simulink model "ponto5"  (R2018a)
settings: Solver=VariableStepAuto  StartTime=0.0  StopTime=100  RelTol=1e-3
values from neighbouring files (symbols this model uses):
  aa0 = 5.27*deg    (= 0.0919788515801)    [tb30.m]
  ah = [xu xw -aa0*u0 -g*cos(tt0) 0 ... (first row only)    [tb30.m]
  bh = [xde xdt; zde 0; mde+mwp*zde mdt; 0 0; 0 0]    [tb30.m]
  deg = pi/180    (= 0.0174532925199)    [tb30.m]
  f = ([1 0 0 0 0;0 0 0 0 1]*g)^-1    [tb30.m]
  ft = 0.3048    [tb30.m]
  k2 = lqr(ah,bh,q,r)    [tb30.m]
  ms = 0.514444444    [tb30.m]
  u0 = 85.4*ms    (= 43.9335555176)    [tb30.m]
libraries: simulink x3
settings Model: Creator=inespassinhas  LastModifiedBy=rafae
settings CodeAppCC: StateflowObjectComments=on

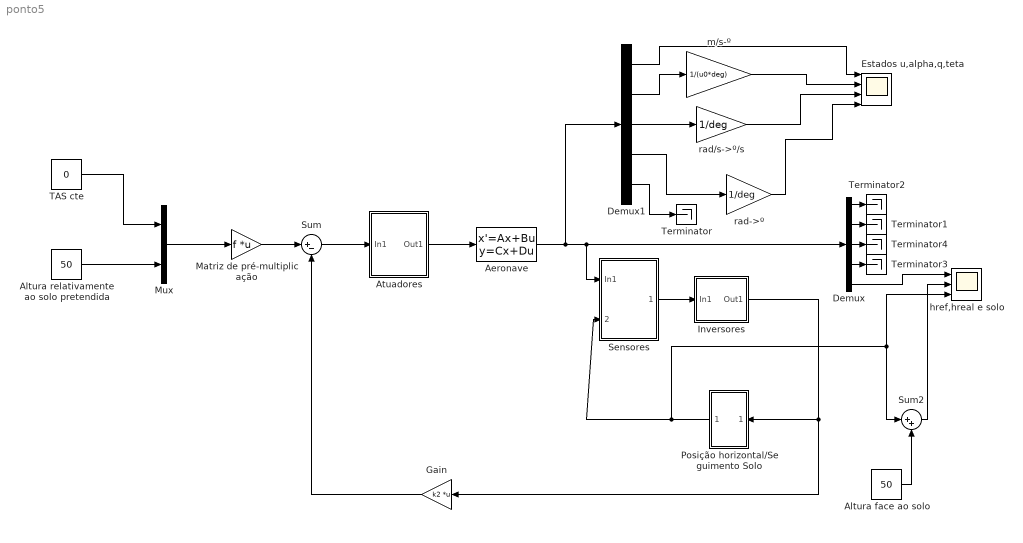
== system ponto5 ==
  Aeronave : StateSpace  A=ah  B=bh  C=eye(5)  D=zeros(5,2)  InitialCondition=[0 0 0 0 50+5*u0]
  "Altura face ao solo   " : Constant  Value=50
  Altura relativamente ao solo pretendida : Constant  Value=50
  Atuadores : Subsystem
  Demux : Demux  Outputs=5
  Demux1 : Demux  Outputs=5
  Estados u,alpha,q,teta : Scope  NumInputPorts=4
  Gain : Gain  Gain=k2  Multiplication=Matrix(K*u)
  Inversores : Subsystem
  Matriz de pré-multiplicação : Gain  Gain=f  Multiplication=Matrix(K*u)
  Mux : Mux  Inputs=2
  Posição horizontal/Seguimento Solo : Subsystem
  Sensores : Subsystem
  Sum : Sum  Inputs=|+-
  Sum2 : Sum  Inputs=|++
  TAS cte : Constant  Value=0
  Terminator{,1..4} (5 alike) : Terminator
  href,hreal e solo : Scope  NumInputPorts=3
  m/s-º : Gain  Gain=1/(u0*deg)
  rad->º : Gain  Gain=1/deg
  rad/s->º/s : Gain  Gain=1/deg
  wires:
  Gain/1 -> Sum/2
  Aeronave/1 -> Sensores/1(In1), Demux/1, Demux1/1
  Mux/1 -> Matriz de pré-multiplicação/1
  Matriz de pré-multiplicação/1 -> Sum/1
  Sensores/1(Out1) -> Inversores/1(In1)
  Atuadores/1(Out1) -> Aeronave/1
  Sum/1 -> Atuadores/1(In1)
  TAS cte/1 -> Mux/1
  Altura relativamente ao solo pretendida/1 -> Mux/2
  Demux/5 -> href,hreal e solo/1
  Sum2/1 -> href,hreal e solo/2
  Inversores/1(Out1) -> Gain/1, Posição horizontal/Seguimento Solo/1(In1)
  Posição horizontal/Seguimento Solo/1(Out1) -> href,hreal e solo/3, Sum2/1, Sensores/2("altura do solo ")
  "Altura face ao solo   "/1 -> Sum2/2
  Demux1/1 -> Estados u,alpha,q,teta/1
  Demux1/2 -> m/s-º/1
  m/s-º/1 -> Estados u,alpha,q,teta/2
  Demux1/3 -> rad/s->º/s/1
  rad/s->º/s/1 -> Estados u,alpha,q,teta/3
  Demux1/4 -> rad->º/1
  rad->º/1 -> Estados u,alpha,q,teta/4
  Demux1/5 -> Terminator/1
  Demux/4 -> Terminator3/1
  Demux/1 -> Terminator2/1
  Demux/2 -> Terminator1/1
  Demux/3 -> Terminator4/1

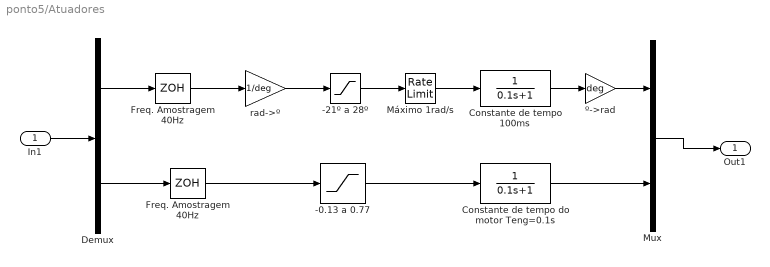
== system ponto5/Atuadores ==
  In1 : Inport
  " Constante de tempo do motor Teng=0.1s" : TransferFcn  Denominator=[0.1 1]
  -0.13 a 0.77 : Saturate  UpperLimit=0.77  LowerLimit=-0.13
  -21º a 28º : Saturate  UpperLimit=28  LowerLimit=-21
  Constante de tempo 100ms : TransferFcn  Denominator=[0.1 1]
  Demux : Demux  Outputs=2
  Freq. Amostragem 40Hz : ZeroOrderHold  SampleTime=1/40
  Freq. Amostragem 40Hz : ZeroOrderHold  SampleTime=1/40
  Mux : Mux  Inputs=2
  Máximo 1rad/s : RateLimiter  RisingSlewLimit=1/deg  FallingSlewLimit=-1/deg  SampleTimeMode=inherited
  rad->º : Gain  Gain=1/deg
  º->rad : Gain  Gain=deg
  Out1 : Outport
  wires:
  Mux/1 -> Out1/1
  In1/1 -> Demux/1
  Demux/2 -> Freq. Amostragem 40Hz/1
  Demux/1 -> Freq. Amostragem 40Hz/1
  Freq. Amostragem 40Hz/1 -> rad->º/1
  rad->º/1 -> -21º a 28º/1
  -21º a 28º/1 -> Máximo 1rad/s/1
  Máximo 1rad/s/1 -> Constante de tempo 100ms/1
  Constante de tempo 100ms/1 -> º->rad/1
  º->rad/1 -> Mux/1
  Freq. Amostragem 40Hz/1 -> -0.13 a 0.77/1
  -0.13 a 0.77/1 -> " Constante de tempo do motor Teng=0.1s"/1
  " Constante de tempo do motor Teng=0.1s"/1 -> Mux/2

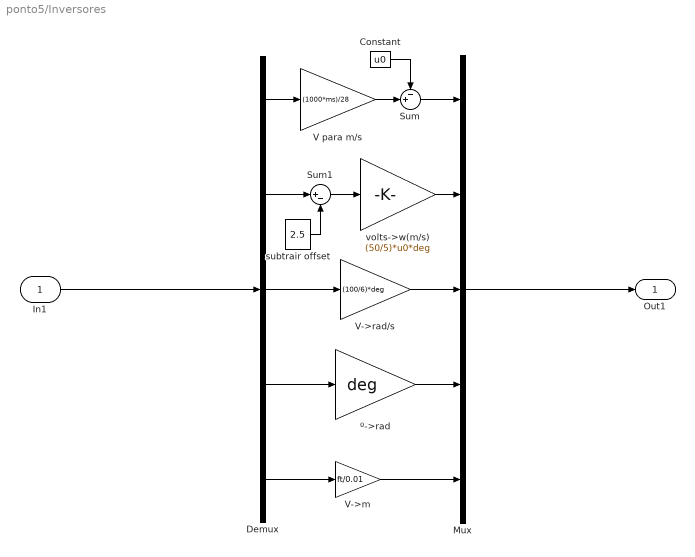
== system ponto5/Inversores ==
  In1 : Inport
  Constant : Constant  Value=u0
  Demux : Demux  Outputs=5
  Mux : Mux  Inputs=5
  Sum : Sum  Inputs=-+|
  Sum1 : Sum  Inputs=|+-
  V para m/s : Gain  Gain=(1000*ms)/28
  V->m : Gain  Gain=ft/0.01
  V->rad/s : Gain  Gain=(100/6)*deg
  subtrair offset : Constant  Value=2.5
  volts->w(m/s) : Gain  Gain=(50/5)*u0*deg
  º->rad : Gain  Gain=deg
  Out1 : Outport
  wires:
  In1/1 -> Demux/1
  Mux/1 -> Out1/1
  Demux/1 -> V para m/s/1
  V para m/s/1 -> Sum/2
  Constant/1 -> Sum/1
  Sum/1 -> Mux/1
  Demux/2 -> Sum1/1
  subtrair offset/1 -> Sum1/2
  Sum1/1 -> volts->w(m/s)/1
  volts->w(m/s)/1 -> Mux/2
  Demux/3 -> V->rad/s/1
  V->rad/s/1 -> Mux/3
  Demux/4 -> º->rad/1
  º->rad/1 -> Mux/4
  Demux/5 -> V->m/1
  V->m/1 -> Mux/5

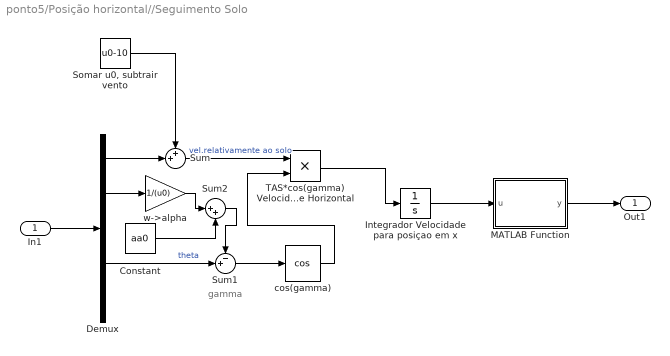
== system ponto5/Posição horizontal//Seguimento Solo ==
  note: gamma
  In1 : Inport
  Constant : Constant  Value=aa0
  Demux : Demux  Outputs=5
  Integrador Velocidade para posiçao em x : Integrator
  MATLAB Function : MATLAB Function  TreatAsAtomicUnit=on
  "Somar u0, subtrair vento" : Constant  Value=u0-10
  Sum : Sum  Inputs=++|
  Sum1 : Sum  Inputs=-+|
  Sum2 : Sum  Inputs=|++
  TAS*cos(gamma) Velocidade Horizontal : Product
  cos(gamma) : Trigonometry  Operator=cos
  w->alpha : Gain  Gain=1/(u0)
  Out1 : Outport
  wires:
  In1/1 -> Demux/1
  Demux/1 -> Sum/2
  "Somar u0, subtrair vento"/1 -> Sum/1
  Demux/2 -> w->alpha/1
  Demux/4 -> Sum1/2  "theta"
  Sum1/1 -> cos(gamma)/1
  cos(gamma)/1 -> TAS*cos(gamma) Velocidade Horizontal/2
  Sum/1 -> TAS*cos(gamma) Velocidade Horizontal/1  "vel.relativamente ao solo"
  TAS*cos(gamma) Velocidade Horizontal/1 -> Integrador Velocidade para posiçao em x/1
  Integrador Velocidade para posiçao em x/1 -> MATLAB Function/1(u)
  MATLAB Function/1(y) -> Out1/1
  Sum2/1 -> Sum1/1
  w->alpha/1 -> Sum2/1
  Constant/1 -> Sum2/2

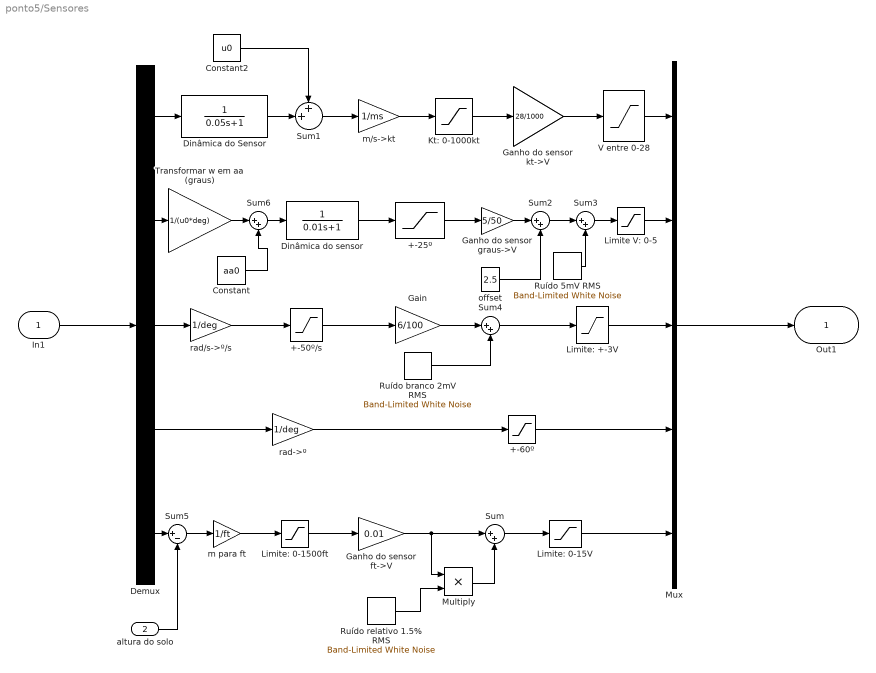
== system ponto5/Sensores ==
  In1 : Inport
  "altura do solo " : Inport  Port=2
  " Dinâmica do Sensor" : TransferFcn  Denominator=[0.05 1]
  +-25º : Saturate  UpperLimit=25  LowerLimit=-25
  +-50º/s : Saturate  UpperLimit=50  LowerLimit=-50
  +-60º : Saturate  UpperLimit=60  LowerLimit=-60
  Constant : Constant  Value=aa0
  Constant2 : Constant  Value=u0
  Demux : Demux  Outputs=5
  Dinâmica do sensor : TransferFcn  Denominator=[0.01 1]
  Gain : Gain  Gain=6/100
  Ganho do sensor ft->V : Gain  Gain=0.01
  Ganho do sensor graus->V : Gain  Gain=5/50
  Ganho do sensor kt->V : Gain  Gain=28/1000
  Kt: 0-1000kt : Saturate  UpperLimit=1000  LowerLimit=0
  Limite V: 0-5 : Saturate  UpperLimit=5  LowerLimit=0
  Limite: +-3V : Saturate  UpperLimit=3  LowerLimit=-3
  Limite: 0-1500ft : Saturate  UpperLimit=1500  LowerLimit=0
  Limite: 0-15V : Saturate  UpperLimit=1500*0.01  LowerLimit=0
  Multiply : Product
  Mux : Mux  Inputs=5
  Ruído 5mV RMS : simulink/Sources/Band-Limited White Noise  Cov=0.005^2/40  Ts=1/40  seed=[23341]
  Ruído branco 2mV RMS : simulink/Sources/Band-Limited White Noise  Cov=(0.002^2)/40  Ts=1/40  seed=[1230]
  Ruído relativo 1.5% RMS : simulink/Sources/Band-Limited White Noise  Cov=(0.015^2)/40  Ts=1/40  seed=[674]
  Sum{,2..4,6} (5 alike) : Sum  Inputs=|++
  Sum1 : Sum  Inputs=++|
  Sum5 : Sum  Inputs=|+-
  Transformar w em aa (graus) : Gain  Gain=1/(u0*deg)
  V entre 0-28 : Saturate  UpperLimit=28  LowerLimit=0
  m para ft : Gain  Gain=1/ft
  m/s->kt : Gain  Gain=1/ms
  offset : Constant  Value=2.5
  rad->º : Gain  Gain=1/deg
  rad/s->º/s : Gain  Gain=1/deg
  Out1 : Outport
  wires:
  In1/1 -> Demux/1
  Mux/1 -> Out1/1
  Demux/2 -> Transformar w em aa (graus)/1
  Dinâmica do sensor/1 -> +-25º/1
  Ganho do sensor ft->V/1 -> Multiply/1, Sum/1
  Demux/1 -> " Dinâmica do Sensor"/1
  Constant2/1 -> Sum1/1
  " Dinâmica do Sensor"/1 -> Sum1/2
  V entre 0-28/1 -> Mux/1
  Ganho do sensor kt->V/1 -> V entre 0-28/1
  +-25º/1 -> Ganho do sensor graus->V/1
  Ganho do sensor graus->V/1 -> Sum2/1
  offset/1 -> Sum2/2
  Limite V: 0-5/1 -> Mux/2
  Sum3/1 -> Limite V: 0-5/1
  Sum2/1 -> Sum3/1
  Ruído 5mV RMS/1 -> Sum3/2
  Demux/3 -> rad/s->º/s/1
  Ruído branco 2mV RMS/1 -> Sum4/2
  Gain/1 -> Sum4/1
  Sum1/1 -> m/s->kt/1
  m/s->kt/1 -> Kt: 0-1000kt/1
  Kt: 0-1000kt/1 -> Ganho do sensor kt->V/1
  rad/s->º/s/1 -> +-50º/s/1
  +-50º/s/1 -> Gain/1
  Sum4/1 -> Limite: +-3V/1
  Limite: +-3V/1 -> Mux/3
  Demux/4 -> rad->º/1
  rad->º/1 -> +-60º/1
  m para ft/1 -> Limite: 0-1500ft/1
  Limite: 0-1500ft/1 -> Ganho do sensor ft->V/1
  Ruído relativo 1.5% RMS/1 -> Multiply/2
  Multiply/1 -> Sum/2
  Sum/1 -> Limite: 0-15V/1
  Limite: 0-15V/1 -> Mux/5
  +-60º/1 -> Mux/4
  Demux/5 -> Sum5/1
  Sum5/1 -> m para ft/1
  "altura do solo "/1 -> Sum5/2
  Transformar w em aa (graus)/1 -> Sum6/1
  Sum6/1 -> Dinâmica do sensor/1
  Constant/1 -> Sum6/2

== matlab function ponto5/Posição horizontal//Seguimento Solo/MATLAB Function ==
  data: u input; y output
function y = fcn(u)

if (u<20*85.4*0.514444444)
   y=(-5/20)*u +5*85.4*0.514444444;
   
elseif (20*85.4*0.514444444<=u) && (u<40*85.4*0.514444444)
   y=0;
   
elseif (40*85.4*0.514444444<=u) && (u<60*85.4*0.514444444)
   %y=2.5*u0*sin((3.14159265359/(20*u0))*u) +2.5*u0;
   y=5*85.4*0.514444444*sin(((u/(20*85.4*0.514444444))-2)*pi/2);

else
    
   y=5*85.4*0.514444444;
end
